simulink model "chap9_4sim"  (R2015a)
settings: Solver=ode45  StartTime=0.0  StopTime=10  RelTol=1e-3
settings Model: Creator=zhr  LastModifiedBy=IT

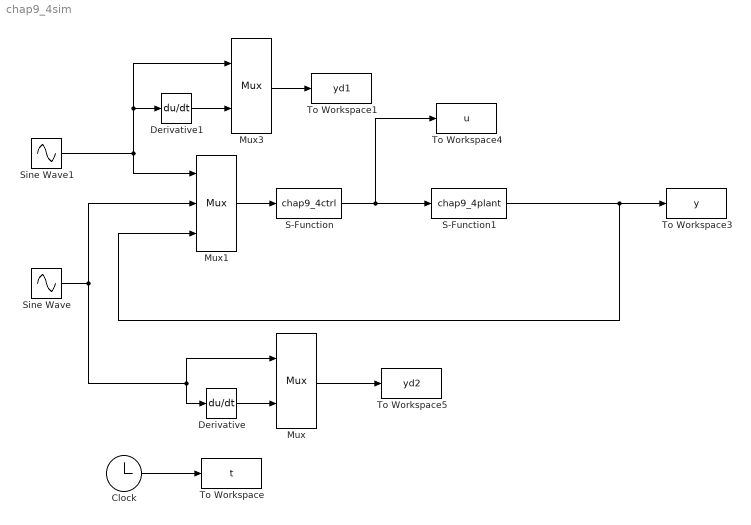
== system chap9_4sim ==
  Clock : Clock
  Derivative : Derivative
  Derivative1 : Derivative
  Mux : Mux  Inputs=2
  Mux1 : Mux  Inputs=3
  Mux3 : Mux  Inputs=2
  S-Function : S-Function  FunctionName=chap9_4ctrl
  S-Function1 : S-Function  FunctionName=chap9_4plant
  Sine Wave : Sin  Amplitude=0.3  SampleTime=0
  Sine Wave1 : Sin  Amplitude=0.3  SampleTime=0
  To Workspace : ToWorkspace  VariableName=t  SampleTime=-1
  To Workspace1 : ToWorkspace  VariableName=yd1  SampleTime=-1
  To Workspace3 : ToWorkspace  VariableName=y  SampleTime=-1
  To Workspace4 : ToWorkspace  VariableName=u  SampleTime=-1
  To Workspace5 : ToWorkspace  VariableName=yd2  SampleTime=-1
  wires:
  Clock/1 -> To Workspace/1
  Sine Wave/1 -> Mux1/2, Derivative/1, Mux/1
  Derivative/1 -> Mux/2
  Mux1/1 -> S-Function/1
  S-Function1/1 -> Mux1/3, To Workspace3/1
  S-Function/1 -> To Workspace4/1, S-Function1/1
  Sine Wave1/1 -> Mux1/1, Derivative1/1, Mux3/1
  Derivative1/1 -> Mux3/2
  Mux3/1 -> To Workspace1/1
  Mux/1 -> To Workspace5/1
